simulink model "IRECSimulink"  (R2024b)
settings: Solver=VariableStepAuto  StartTime=0.0  StopTime=30  RelTol=1e-3
PreLoadFcn:
  | setup_initials
InitFcn:
  | % ---- Simulation constants ----
  | V_sim_start   = 332;
  | altitude_initial = 6088;
  | mass_burnout  = 18.2;
  | 
  | % ---- Locate CSV next to the model file ----
  | mdlFile = get_param(bdroot, 'FileName');     % full path to the .slx
  | mdlDir  = fileparts(mdlFile);
  | csvName = 'MachNumberCDMap.csv';
  | csvPath = fullfile(mdlDir, csvName);
  | 
  | assert(isfile(csvPath), ...
  |     "Can't find %s. Put it in the same folder as the model or update csvPath.", csvPath);
  | 
  | % ---- Read CSV (robust to column name casing) ----
  | T = readtable(csvPath);
  | 
  | % Try common header names; fall back to first two columns
  | varNamesLower = lower(string(T.Properties.VariableNames));
  | ixM = find(varNamesLower == "machnumber" | varNamesLower == "mach", 1);
  | ixC = find(varNamesLower == "cd" | varNamesLower == "drag" | varNamesLower == "dragcoefficient", 1);
  | 
  | if isempty(ixM) || isempty(ixC)
  |     % assume first two columns are Mach, Cd
  |     ixM = 1; ixC = 2;
  | end
  | 
  | mach = T{:, ixM};
  | cd   = T{:, ixC};
  | 
  | % ---- Clean & sort (required for lookup tables) ----
  | valid = ~(isnan(mach) | isnan(cd));
  | mach = mach(valid);
  | cd   = cd(valid);
  | 
  | % ensure strictly ascending & unique breakpoints
  | [mach, idx] = sort(mach(:));
  | cd = cd(idx);
  | [mach, uniqIdx] = unique(mach, 'stable');
  | cd = cd(uniqIdx);
  | 
  | % OPTIONAL: clamp or warn if too few points
  | assert(numel(mach) >= 2, 'Need at least two (Mach, Cd) points for 1-D interpolation.');
  | 
  | % ---- Now point your 1-D Lookup Table block at these variables ----
  | % Breakpoints (x): mach
  | % Table data   (y): cd
  | % Interp: 'Linear' (or 'PCHIP'); Extrap: 'Clip' (recommended)
model workspace (MAT data in the model file):
  Cd_body = 0.733
  Sig = Simulink.Signal
  Sig.Dimensions = -1
  Sig.DimensionsMode = 'auto'
  Sig.Complexity = 'auto'
  Sig.SampleTime = -1
  Sig.SamplingMode = 'auto'
  Sig.DataType = 'auto'
  V_initial = 0
  Var = 0
  mass = 0.964
settings Model: Creator=lawtonskaling  LastModifiedBy=lawtonskaling

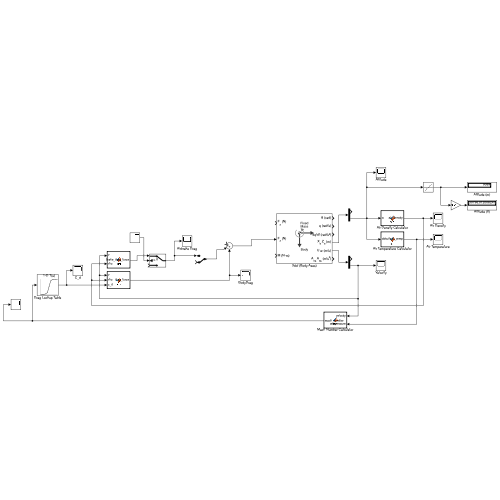
[thumbnail: Simulink's stored preview of the top-level diagram]
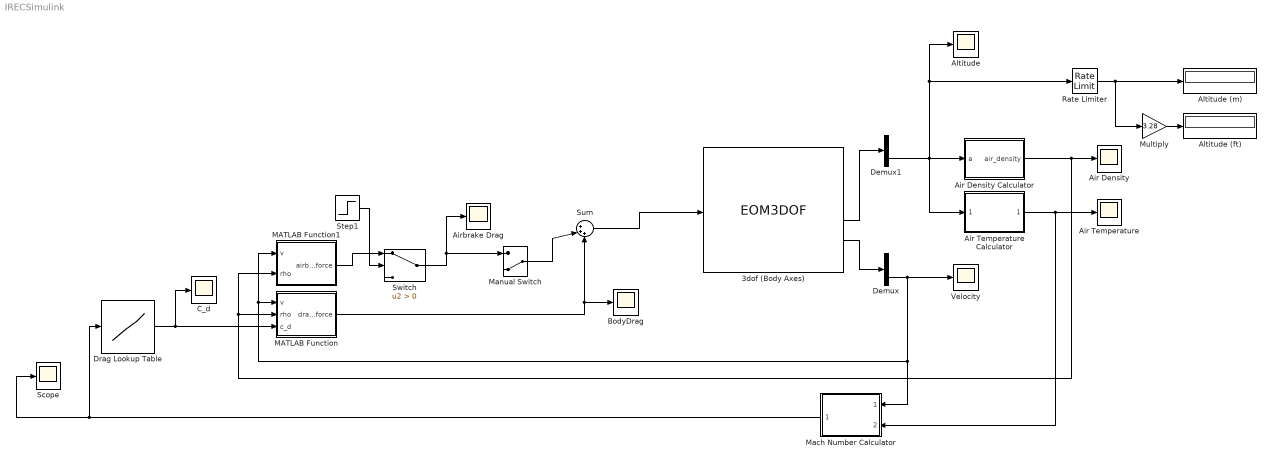
== system IRECSimulink ==
  3dof (Body Axes) : EOM3DOF  v_ini=V_sim_start  alpha_ini=90  pos_ini=[0 altitude_initial]  mass=mass_burnout  g=-9.81
  Air Density : Scope
  Air Density Calculator : MATLAB Function  TreatAsAtomicUnit=on
  Air Temperature : Scope
  Air Temperature Calculator : MATLAB Function  TreatAsAtomicUnit=on
  Airbrake Drag : Scope
  Altitude : Scope
  Altitude (ft) : Display
      settings: Decimation=3
  Altitude (m) : Display
  BodyDrag : Scope
  C_d : Scope
  Demux : Demux  Outputs=2
  Demux1 : Demux  Outputs=2
  Drag Lookup Table : Lookup_n-D  NumberOfTableDimensions=1  BreakpointsForDimension1=mach  Table=cd  ExtrapMethod=Clip  InternalRulePriority=Speed  RndMeth=Simplest
  MATLAB Function : MATLAB Function  TreatAsAtomicUnit=on
  MATLAB Function1 : MATLAB Function  TreatAsAtomicUnit=on
  Mach Number Calculator : MATLAB Function  TreatAsAtomicUnit=on
  Manual Switch : ManualSwitch  CurrentSetting=0
  Multiply : Gain  Gain=3.28
  Rate Limiter : RateLimiter  RisingSlewLimit=inf  FallingSlewLimit=0  SampleTimeMode=inherited
  Scope : Scope
  Step1 : Step  SampleTime=0
  Sum : Sum  Inputs=|+++
  Switch : Switch  Criteria=u2 > Threshold  SaturateOnIntegerOverflow=off  InputSameDT=off
  Velocity : Scope
  wires:
  Sum/1 -> 3dof (Body Axes)/2
  MATLAB Function/1(drag_force) -> Sum/3, BodyDrag/1
  3dof (Body Axes)/5 -> Demux/1
  Demux/2 -> Velocity/1, Mach Number Calculator/1(velocity), MATLAB Function1/1(v), MATLAB Function/1(v)
  3dof (Body Axes)/4 -> Demux1/1
  Demux1/2 -> Air Temperature Calculator/1(altitude), Altitude/1, Rate Limiter/1, Air Density Calculator/1(a)
  Rate Limiter/1 -> Multiply/1, Altitude (m)/1
  Manual Switch/1 -> Sum/2
  Switch/1 -> Manual Switch/1, Airbrake Drag/1
  Step1/1 -> Switch/2
  MATLAB Function1/1(airbrake_drag_force) -> Switch/1
  Air Density Calculator/1(air_density) -> MATLAB Function1/2(rho), MATLAB Function/2(rho), Air Density/1
  Drag Lookup Table/1 -> C_d/1, MATLAB Function/3(c_d)
  Mach Number Calculator/1(mach_number) -> Scope/1, Drag Lookup Table/1
  Air Temperature Calculator/1(air_temp) -> Mach Number Calculator/2(temperature), Air Temperature/1
  Multiply/1 -> Altitude (ft)/1

== matlab function IRECSimulink/MATLAB Function1 ==
  data: v input; airbrake_drag_force output; rho input
function airbrake_drag_force = fcn(v, rho)

%A_ref = (3 * 25 * 30)/1000^2; %Shasta
A_ref = (4 * 50 * 60)/1000^2;
c_d = 1.5;

body_drag = 0.5*rho*v.^2*c_d*A_ref;

airbrake_drag_force = body_drag .* sign(v) * -1;

== matlab function IRECSimulink/MATLAB Function ==
  data: v input; drag_force output; rho input; c_d input
function drag_force = fcn(v, rho, c_d)

%rho = 0.59; %kg / m^3
% A_ref = 3505 / 1000^2;% Shasta
% c_d = 0.733; % Shasta

%c_d = 0.644; %IREC
A_ref = 8107 / 1000^2; %IREC

body_drag = 0.5*rho*v.^2*c_d*A_ref;

drag_force = body_drag .* sign(v) * -1;

== matlab function IRECSimulink/Air Density Calculator ==
  data: a input; air_density output
function air_density = fcn(a)

air_density_ground = 1.22;
air_density_30000 = 0.46;

air_density = air_density_ground - (air_density_ground-air_density_30000)*a/9144;

== matlab function IRECSimulink/Mach Number Calculator ==
  data: velocity input; mach_number output; temperature input
function mach_number = fcn(velocity, temperature)

gamma = 1.4;
R = 287.05;

mach_number = velocity / sqrt(gamma * R * (temperature+273));

== matlab function IRECSimulink/Air Temperature Calculator ==
  data: altitude input; air_temp output
function air_temp = fcn(altitude)

air_temp_ground = 15;
air_temp_9000 = -44;

air_temp = air_temp_ground - (air_temp_ground-air_temp_9000)*altitude/9000;
